simulink model "ProjectSimulink"  (R2023a)
settings: Solver=VariableStepAuto  StartTime=0.0  StopTime=10  RelTol=1e-3
values from neighbouring files (symbols this model uses):
  b1 = 0.25    [ProjectAStateSpaceData.m]    (also in ProjectSimulinkData.m)
  b2 = 0.15    [ProjectAStateSpaceData.m]    (also in ProjectSimulinkData.m)
  F = 0.15    [ProjectSimulinkData.m]
  k1 = 8    [ProjectAStateSpaceData.m]    (also in ProjectSimulinkData.m)
  k2 = 6    [ProjectAStateSpaceData.m]    (also in ProjectSimulinkData.m)
  k3 = 6    [ProjectAStateSpaceData.m]    (also in ProjectSimulinkData.m)
  k4 = 5    [ProjectAStateSpaceData.m]    (also in ProjectSimulinkData.m)
  m1 = 0.2    [ProjectAStateSpaceData.m]    (also in ProjectSimulinkData.m)
  m2 = 0.15    [ProjectAStateSpaceData.m]    (also in ProjectSimulinkData.m)
  m3 = 0.1    [ProjectAStateSpaceData.m]    (also in ProjectSimulinkData.m)
settings Model: Creator=student352en  LastModifiedBy=ess
settings SolverCC: AlgebraicLoopSolver=TrustRegion
settings DebuggingCC: UnconnectedInputMsg=warning  UnconnectedOutputMsg=warning  UnconnectedLineMsg=warning
settings ModelReferenceCC: EnableRefExpFcnMdlSchedulingChecks=on

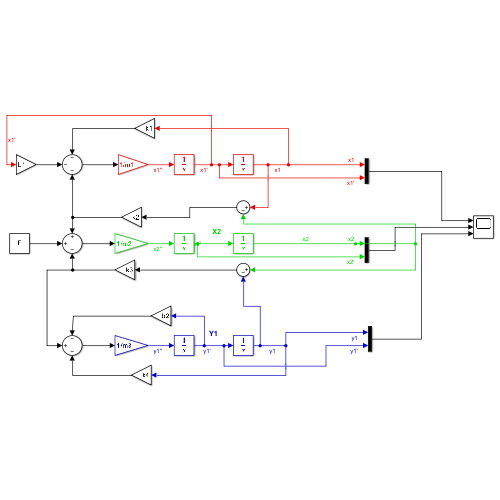
[thumbnail: Simulink's stored preview of the top-level diagram]
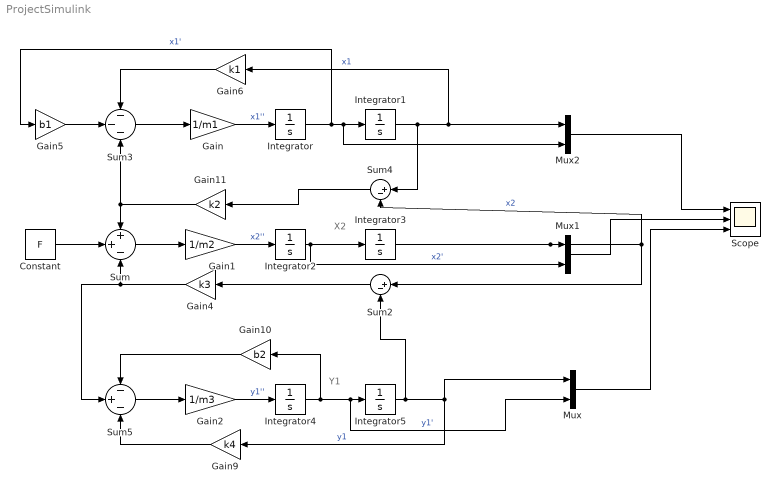
== system ProjectSimulink ==
  note: Y1
  note: X2
  Constant : Constant  Value=F  SampleTime=0.01
  Gain : Gain  Gain=1/m1
  Gain1 : Gain  Gain=1/m2
  Gain10 : Gain  Gain=b2
  Gain11 : Gain  Gain=k2
  Gain2 : Gain  Gain=1/m3
  Gain4 : Gain  Gain=k3
  Gain5 : Gain  Gain=b1
  Gain6 : Gain  Gain=k1
  Gain9 : Gain  Gain=k4
  Integrator{,1..5} (6 alike) : Integrator
  Mux : Mux  Inputs=2
  Mux1 : Mux  Inputs=2
  Mux2 : Mux  Inputs=2
  Scope : Scope  NumInputPorts=3
  Sum : Sum  Inputs=++-
  Sum2 : Sum  Inputs=|+-
  Sum3 : Sum  Inputs=---
  Sum4 : Sum  Inputs=|+-
  Sum5 : Sum  Inputs=-+-
  wires:
  Integrator/1 -> Mux2/2, Integrator1/1, Gain5/1  "x1'"
  Integrator2/1 -> Mux1/2, Integrator3/1  "x2'"
  Integrator4/1 -> Gain10/1, Mux/2, Integrator5/1  "y1'"
  Gain/1 -> Integrator/1  "x1''"
  Gain1/1 -> Integrator2/1  "x2''"
  Gain2/1 -> Integrator4/1  "y1''"
  Integrator1/1 -> Sum4/1, Mux2/1, Gain6/1  "x1"
  Integrator5/1 -> Mux/1, Gain9/1, Sum2/2  "y1"
  Constant/1 -> Sum/2
  Sum/1 -> Gain1/1
  Integrator3/1 -> Sum2/1, Sum4/2, Mux1/1  "x2"
  Sum2/1 -> Gain4/1
  Gain4/1 -> Sum/3, Sum5/2
  Gain5/1 -> Sum3/2
  Sum3/1 -> Gain/1
  Gain6/1 -> Sum3/1
  Sum4/1 -> Gain11/1
  Sum5/1 -> Gain2/1
  Gain9/1 -> Sum5/3
  Gain10/1 -> Sum5/1
  Gain11/1 -> Sum/1, Sum3/3
  Mux/1 -> Scope/3
  Mux1/1 -> Scope/2
  Mux2/1 -> Scope/1
